simulink model "PMSM_Arch"  (R2022b)
settings: Solver=FixedStepDiscrete  StartTime=0.0  StopTime=10.0  RelTol=1e-3
settings Model: Creator=MAAM  LastModifiedBy=MAAM

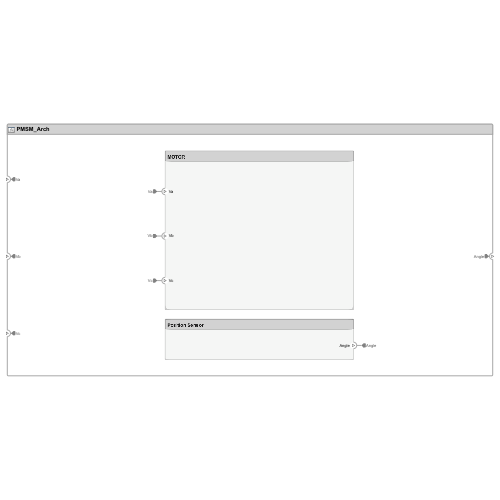
[thumbnail: Simulink's stored preview of the top-level diagram]
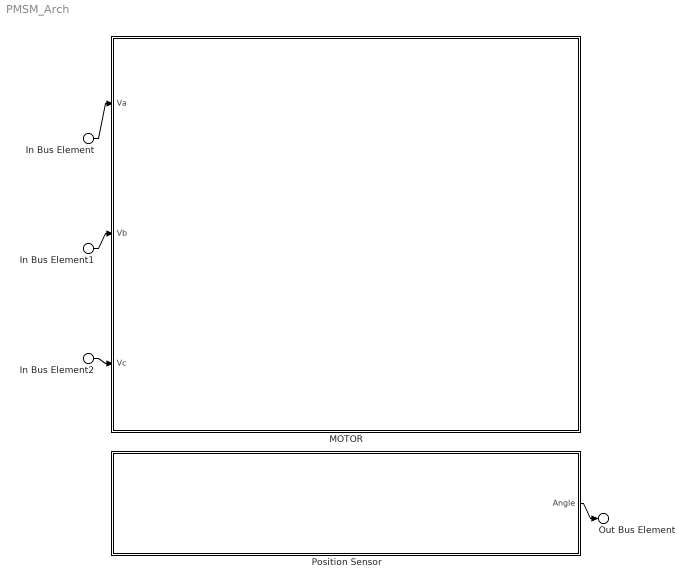
== system PMSM_Arch ==
  In Bus Element : Inport  PortName=Va
  In Bus Element1 : Inport  Port=2  PortName=Vb
  In Bus Element2 : Inport  Port=3  PortName=Vc
  MOTOR : Subsystem
      settings: PortSchema="{\"entries\":[{\"content\":{\"headerSize\":26,\"margin\":15,\"minimumSpacing\":25,\"sides\":[{\"content\":{\"connectorIds\":[\"In1\",\"In2\",\"In3\"]},\"type\":\"ConnectorPlacement.EquallySpacedRectSide\",\"uuid\":\"ecb73a61-b18a-4e6f-9a16-a7412467d3dc\"},{\"content\":{\"connectorIds\":[],\"side\":\"RIGHT\"},\"type\":\"ConnectorPlacement.EquallySpacedRectSide\",\"uuid\":\"05d75da6-23d5-4864-9569-f2b0c11a82bb\"},{\"content\":{\"connectorIds\":[],\"side\":\"TOP\"},\"type\":\"ConnectorPlacement.EquallySpacedRectSide\",\"uuid\":\"f7c561b3-9491-4c59-9ccb-7eaec9c6a3d8\"}]},\"type\":\"ConnectorPlacement.EquallySpacedConnector\",\"uuid\":\"7fcac072-6609-4f2b-820d-d62cc0efbf31\"}],\"packageUris\":[\"http://schema.mathworks.com/mf0/Connector/R2020b\"],\"version\":\"1.0\"}"
  Position Sensor : Subsystem
      settings: PortSchema="{\"entries\":[{\"content\":{\"headerSize\":26,\"margin\":15,\"minimumSpacing\":25,\"sides\":[{\"content\":{\"connectorIds\":[]},\"type\":\"ConnectorPlacement.EquallySpacedRectSide\",\"uuid\":\"ecb73a61-b18a-4e6f-9a16-a7412467d3dc\"},{\"content\":{\"connectorIds\":[\"Out1\"],\"side\":\"RIGHT\"},\"type\":\"ConnectorPlacement.EquallySpacedRectSide\",\"uuid\":\"05d75da6-23d5-4864-9569-f2b0c11a82bb\"},{\"content\":{\"connectorIds\":[],\"side\":\"TOP\"},\"type\":\"ConnectorPlacement.EquallySpacedRectSide\",\"uuid\":\"f7c561b3-9491-4c59-9ccb-7eaec9c6a3d8\"}]},\"type\":\"ConnectorPlacement.EquallySpacedConnector\",\"uuid\":\"7fcac072-6609-4f2b-820d-d62cc0efbf31\"}],\"packageUris\":[\"http://schema.mathworks.com/mf0/Connector/R2020b\"],\"version\":\"1.0\"}"
  Out Bus Element : Outport  PortName=Angle
  wires:
  In Bus Element/1 -> MOTOR/1(Va)
  In Bus Element1/1 -> MOTOR/2(Vb)
  In Bus Element2/1 -> MOTOR/3(Vc)
  Position Sensor/1(Angle) -> Out Bus Element/1

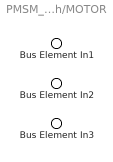
== system PMSM_Arch/MOTOR ==
  Bus Element In1 : Inport  PortName=Va
  Bus Element In2 : Inport  Port=2  PortName=Vb
  Bus Element In3 : Inport  Port=3  PortName=Vc

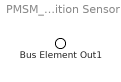
== system PMSM_Arch/Position Sensor ==
  Bus Element Out1 : Outport  PortName=Angle
